simulink model "Ambient_temp_individual"  (R2024b)
settings: Solver=ode45  StartTime=0.0  StopTime=86400*365  MaxStep=1e4  RelTol=1e-3
values from neighbouring files (symbols this model uses):
  SummerDay = 31    [IDP3_Control_System.m]
  SummerNight = 25    [IDP3_Control_System.m]
  WinterDay = 32    [IDP3_Control_System.m]
  WinterNight = 26    [IDP3_Control_System.m]
libraries: slpidlib x1
settings Model: Creator=User  LastModifiedBy=User

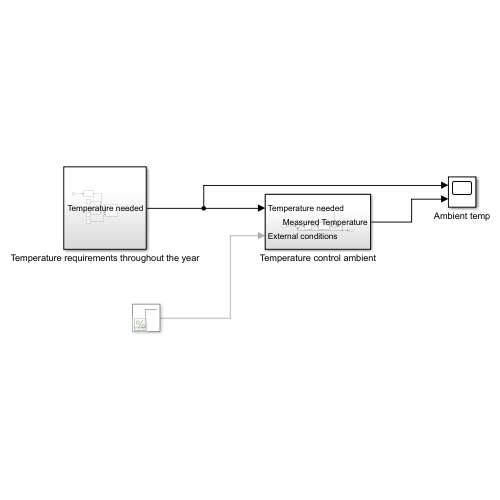
[thumbnail: Simulink's stored preview of the top-level diagram]
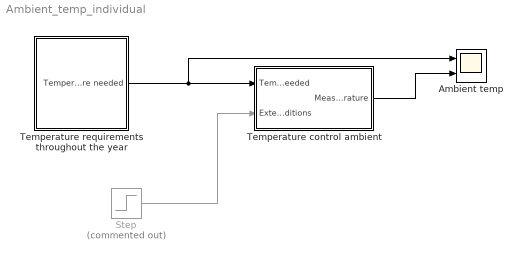
== system Ambient_temp_individual ==
  Ambient temp : Scope  NumInputPorts=2
  Step : Step  Commented=on  Time=4e4  After=10  SampleTime=0
  Temperature control ambient : Subsystem
  Temperature requirements throughout the year : Subsystem
  wires:
  Temperature requirements throughout the year/1(Temperature needed) -> Ambient temp/1, Temperature control ambient/1(Temperature needed)
  Temperature control ambient/1(Measured Temperature) -> Ambient temp/2
  Step/1 -> Temperature control ambient/2(External conditions)

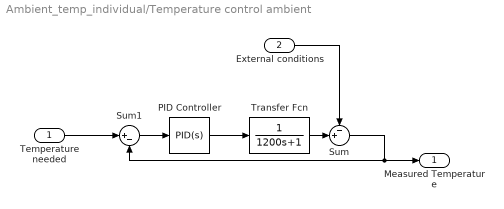
== system Ambient_temp_individual/Temperature control ambient ==
  Temperature needed : Inport
  External conditions : Inport  Port=2
  PID Controller : slpidlib/PID Controller  Controller=PID  Form=Parallel  TimeDomain=Continuous-time  UseExternalTs=off  SampleTime=-1  IntegratorMethod=Forward Euler  FilterMethod=Forward Euler  ControllerParametersSource=internal  P=200  I=0.5  UseKiTs=off  D=0  UseExternalDerivativeSource=off  N=100  UseFilter=on  TunerSelectOption=Transfer Function Based (PID Tuner App)  InitialConditionSource=internal  InitialConditionForIntegrator=0  InitialConditionForFilter=0  DifferentiatorICPrevScaledInput=0  ExternalReset=none  TrackingMode=off  Kt=1  LimitOutput=off  SatLimitsSource=internal  UpperSaturationLimit=inf  LowerSaturationLimit=-inf  LinearizeAsGain=on  AntiWindupMode=none  Kb=1  LimitIntegrator=off  UpperIntegratorSaturationLimit=inf  LowerIntegratorSaturationLimit=-inf  POutMin=[]  POutMax=[]  IOutMin=[]  IOutMax=[]  DOutMin=[]  DOutMax=[]  NOutMin=[]  NOutMax=[]  SumOutMin=[]  SumOutMax=[]  SaturationOutMin=[]  SaturationOutMax=[]  PParamMin=[]  PParamMax=[]  IParamMin=[]  IParamMax=[]  DParamMin=[]  DParamMax=[]  NParamMin=[]  NParamMax=[]  KbParamMin=[]  KbParamMax=[]  KtParamMin=[]  KtParamMax=[]  KbOutMin=[]  KbOutMax=[]  KtOutMin=[]  KtOutMax=[]  IntegratorOutMin=[]  IntegratorOutMax=[]  FilterOutMin=[]  FilterOutMax=[]  SumI1OutMin=[]  SumI1OutMax=[]  SumI2OutMin=[]  SumI2OutMax=[]  SumI3OutMin=[]  SumI3OutMax=[]  SumI4OutMin=[]  SumI4OutMax=[]  SumDOutMin=[]  SumDOutMax=[]  DifferentiatorOutMin=[]  DifferentiatorOutMax=[]  FilterDiffOutCoefMin=[]  FilterDiffOutCoefMax=[]  ReciprocalOutMin=[]  ReciprocalOutMax=[]  SumDenOutMin=[]  SumDenOutMax=[]  SumNumOutMin=[]  SumNumOutMax=[]  DivideOutMin=[]  DivideOutMax=[]  UdiffTsProdOutMin=[]  UdiffTsProdOutMax=[]  NTsProdOutMin=[]  NTsProdOutMax=[]  UintegralTsProdOutMin=[]  UintegralTsProdOutMax=[]  UngainTsProdOutMin=[]  UngainTsProdOutMax=[]  ClampingZeroOutDataTypeStr=Inherit: Inherit via back propagation  ClampingZeroOutMin=[]  ClampingZeroOutMax=[]  FilterDenConstantOutDataTypeStr=Inherit: Inherit via back propagation  FilterDenConstantOutMin=[]  FilterDenConstantOutMax=[]  PCopyOutDataTypeStr=Inherit: Inherit via back propagation  PCopyOutMin=[]  PCopyOutMax=[]  NCopyOutDataTypeStr=Inherit: Inherit via back propagation  NCopyOutMin=[]  NCopyOutMax=[]  IntegratorContinuousStateAttributes=''  IntegratorStateMustResolveToSignalObject=off  IntegratorRTWStateStorageClass=Auto  FilterContinuousStateAttributes=''  FilterStateMustResolveToSignalObject=off  FilterRTWStateStorageClass=Auto  ParallelPVariant=InternalParameters  IdealPVariant=Disabled  IVariant=InternalParameters  DVariant=InternalParameters  IntegratorVariant=Continuous  SatVariant=Disabled  AWVariant=Passthrough  PCopyVariant=Disabled  TRVariant=Disabled  FdbkBlocksVariant=Forward  IdealPFdbkVariant=Disabled  SatFdbkVariant=Disabled  DerivativeFilterVariant=ContFilter  NVariant=InternalParameters  NCopyVariant=Disabled  FilterICVariant=InternalICsFilter  IntegratorICVariant=InternalICs  ExternalResetVariant=Disabled  TRSumVariant=Passthrough  SumFdbkVariant=Disabled  SumVariant=Sum_PID  TsampFilterVariant=InternalTs  TsampNgainVariant=Passthrough  TsampIntegralVariant=Disabled_SignalSpec  ExternalSaturationOutDataTypeStr=Inherit: Same as second input  DerivativeSourceVariant=ErrorSignal  PreIntVariant=InternalPreInt
  Sum : Sum  Inputs=-+|
  Sum1 : Sum  Inputs=|+-
  Transfer Fcn : TransferFcn  Denominator=[1200 1]
  Measured Temperature : Outport
  wires:
  Sum1/1 -> PID Controller/1
  Temperature needed/1 -> Sum1/1
  PID Controller/1 -> Transfer Fcn/1
  Transfer Fcn/1 -> Sum/2
  Sum/1 -> Sum1/2, Measured Temperature/1
  External conditions/1 -> Sum/1

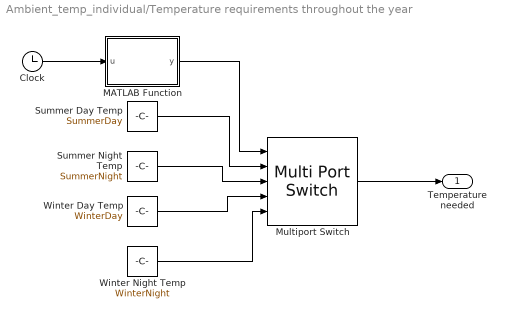
== system Ambient_temp_individual/Temperature requirements throughout the year ==
  Clock : Clock
  MATLAB Function : MATLAB Function  TreatAsAtomicUnit=on
  Multiport Switch : MultiPortSwitch  Inputs=4  SaturateOnIntegerOverflow=off  InputSameDT=off
  Summer Day Temp : Constant  Value=SummerDay
  Summer Night Temp : Constant  Value=SummerNight
  Winter Day Temp : Constant  Value=WinterDay
  Winter Night Temp : Constant  Value=WinterNight
  Temperature needed : Outport
  wires:
  Multiport Switch/1 -> Temperature needed/1
  Clock/1 -> MATLAB Function/1(u)
  Summer Day Temp/1 -> Multiport Switch/2
  Summer Night Temp/1 -> Multiport Switch/3
  Winter Day Temp/1 -> Multiport Switch/4
  Winter Night Temp/1 -> Multiport Switch/5
  MATLAB Function/1(y) -> Multiport Switch/1

== matlab function Ambient_temp_individual/Temperature requirements throughout the year/MATLAB Function ==
  settings: updateMethod=DISCRETE
  data: u input; y output
function y = fcn(u)
    persistent rDaily rSeason; 
   
    if isempty(rDaily)
        rDaily = 0;
    end
    if isempty(rSeason)
        rSeason = 0;
    end
    
    % Extract time components
    TDaily = u - rDaily * 24 * 60 * 60;  % Time since last daily reset
    TSeason = u - rSeason * 365 * 24 * 60 * 60;  % Time since last yearly reset
    
    % Check if a new day has passed
    if TDaily >= 24 * 60 * 60
        rDaily = rDaily + 1;
        TDaily = TDaily - 24 * 60 * 60;  % Reset daily counter
    end
    
    % Check if a new year has passed
    if TSeason >= 365 * 24 * 60 * 60
        rSeason = rSeason + 1;
        TSeason = TSeason - 365 * 24 * 60 * 60;  % Reset yearly counter
    end
    
    % Determine if it's day (6 AM to 6 PM)
    IsDay = (TDaily >= 6 * 60 * 60) && (TDaily < 18 * 60 * 60);
    IsNight = ~IsDay;
    
    % Determine season 
    summerStart = (31 + 28 + 31) * 24 * 60 * 60;  % April 1st
    summerEnd = summerStart + (30 + 31 + 30 + 31 + 31 + 30) * 24 * 60 * 60;  % September  30th
    
    IsSummer = (TSeason >= summerStart) && (TSeason <= summerEnd);
    IsWinter = ~IsSummer; 
    % Assign output based on season and time of day
    if IsSummer && IsDay
        y = 1;  % Summer, Day
    elseif IsSummer && IsNight
        y = 2;  % Summer, Night
    elseif IsWinter && IsDay
        y = 3;  % Winter, Day
    else
        y = 4;  % Winter, Night
    end
end
